simulink library "dspindex"  (Simulink 5.0)
libraries: dspmtrx3 x3
settings Model: RequirementInfo=9  CovMetricSettings=d  Creator=don  LastModifiedBy=mkhan  ExtModeAutoUpdateStatusClock=off  TargetHWChar=2  TargetHWWordLengths=8,16,32,32

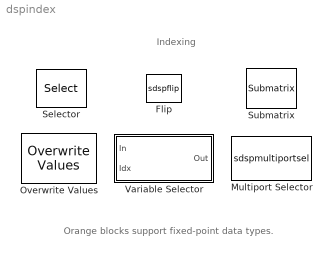
== system dspindex ==
  note: Indexing
  note: Orange blocks support fixed-point data types.
  Flip : S-Function  FunctionName=sdspflip  Parameters=dim  mask(Flip){dim=Columns}
      mask prompts: dim "Flip along:"
      mask help: Reverse order of vector elements. For oriented inputs, reverse the order along the specified dimension.
      settings: CopyFcn=dspfixptcopycallback
      mask Help: web(dspbhelp);
      mask StyleString: popup(Rows|Columns)
      mask Display: plot(0,0,100,100,[47 40 40 47],[20 20 90 90],[53 60 60 53],[90 90 20 20],[75 76 81 80 73],[34 24 40 60 90],[83 76],[29 24],[19 30 19 19 26],[86 84 72 50 20],[29 30],[71 84])
  Multiport Selector : S-Function  FunctionName=sdspmultiportsel  Parameters=rowsOrCols, numOutports, flatIdxVect, flatLenVect, idxErrMode  mask(Multiport Selector){rowsOrCols=Rows, idxCellArray={ 4, [1:2 5], [7; 8], 10:-1:6 }, idxErrMode=Clip Index}
      mask prompts: rowsOrCols "Select:"; idxCellArray "Indices to output:"; idxErrMode "Invalid index:"
      mask help: Output specified rows or columns to one or more output ports. The number of output ports is determined by the number of index vectors, each specified as a separate vector entry in a cell array. Indices are 1-based and need not be unique.
      mask init:
      | [numOutports, flatLenVect, flatIdxVect] = dspblkmultiportsel(idxCellArray);
      settings: CopyFcn=dspfixptcopycallback
      mask Help: web(dspbhelp);
      mask StyleString: popup(Rows|Columns),edit,popup(Clip Index|Clip and Warn|Generate Error)
      mask Display: disp(['Select\n' &1]);
  Overwrite Values : dspmtrx3/Overwrite Values  OverWriteDiag=Submatrix  valFrom2ndIP=Specify via dialog  ConstValue=0  RowSpan=Range of rows  RowStartMode=First  RowStartIndex=1  RowEndMode=Last  RowEndIndex=1  ColSpan=Range of columns  ColStartMode=First  ColStartIndex=1  ColEndMode=Last  ColEndIndex=1  DiagSpan=Range of elements  DiagStartMode=Index  DiagStartIndex=2  DiagEndMode=Index  DiagEndIndex=4
  Selector : Selector  Elements=[1 3]  InputPortWidth=3
      settings: CopyFcn=dspfixptcopycallback
  Submatrix : dspmtrx3/Submatrix  RowSpan=Range of rows  RowStartMode=First  RowStartIndex=1  RowEndMode=Last  RowEndIndex=1  ColSpan=Range of columns  ColStartMode=First  ColStartIndex=1  ColEndMode=Last  ColEndIndex=1
  Variable Selector : Subsystem  mask(Variable Selector){rowsOrCols=Rows, IdxMode=Variable, Elements=[1 3], ZerOneIdxMode=One-based, errmode=Clip Index}
      mask prompts: rowsOrCols "Select:"; IdxMode "Selector mode:"; ZerOneIdxMode "Index mode:"; errmode "Invalid index:"
      mask help: Selects and/or reorders the rows or columns of the input according to a specified vector of indices (the indices need not be unique). The 'Selector mode' parameter determines whether the block uses the same indices for every input ('Fixed'), or uses different indices for every input ('Variable'). When set to 'Variable', you provide the vector of indices through an input port.
      mask init:
      | dspblkvarsel2('init');
      settings: CopyFcn=dspfixptcopycallback
      mask Help: web(dspbhelp);
      mask StyleString: popup(Rows|Columns),popup(Fixed|Variable),edit,popup(Zero-based|One-based),popup(Clip Index|Clip and Warn|Generate Error)
      mask CallbackString: dspblkvarsel2|dspblkvarsel2||dspblkvarsel2|
      mask Display: disp(['Select\n' &1]);

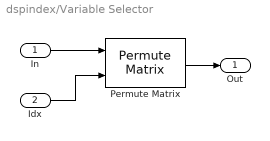
== system dspindex/Variable Selector ==
  In : Inport
  Idx : Inport  Port=2
  Permute Matrix : dspmtrx3/Permute Matrix  mode=Rows  ZeroOneIdxMode=One-based  errmode=Clip Index  checkDims=off
  Out : Outport
  wires:
  In/1 -> Permute Matrix/1
  Permute Matrix/1 -> Out/1
  Idx/1 -> Permute Matrix/2
